simulink model "Speed_Controller"  (R2019b)
settings: Solver=VariableStepAuto  StartTime=0.0  StopTime=10.0  RelTol=1e-3
values from neighbouring files (symbols this model uses):
  B = 1/3*Te_n*1/w_b    (= 1.3022339824)    [tram.m]
  e_n = Ks*ie_max*w_b    (= 540)    [tram.m]
  g = 9.81    [tram.m]
  ie_max = 1    [tram.m]
  J = m_t*r_whl^2    (= 73.2506615098)    [tram.m]
  kb_e = 1/tau_e    (= 1)    [tram.m]
  kb_spd = 1/tau_s    (= 5)    [tram.m]
  Kie = Ci_e.Ki    [tram.m]
  Kim = Cm.Ki    [tram.m]
  Kpe = Ci_e.Kp    [tram.m]
  Kpm = Cm.Kp    [tram.m]
  Ks = v_line*eta/(ie_max*w_b)    (= 1.71974522293)    [tram.m]
  Le = tau_e*Re    (= 120)    [tram.m]
  m_t = m_train + m_load    (= 26000)    [tram.m]
  r_whl = s_b/w_b*10/36    (= 0.0530785562633)    [tram.m]
  Re = ve_max/ie_max    (= 120)    [tram.m]
  w_b = 314    [tram.m]
undefined symbols (not defined in the file or in its folder): sigbuilder_block
settings Model: Creator=hassancurrimbhoy  LastModifiedBy=hassancurrimbhoy

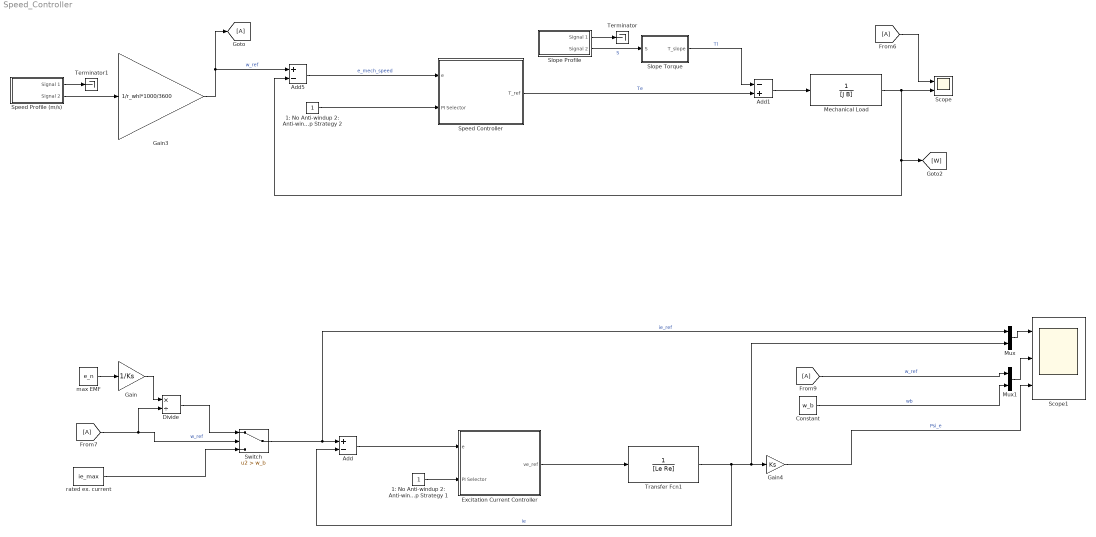
== system Speed_Controller ==
  1: No Anti-windup 2: Anti-windup Stragtegy 1 3: Anti-windup Strategy 2 : Constant
  1: No Anti-windup 2: Anti-windup Strategy 1 3: Anti-windup Strategy 1 : Constant
  Add : Sum  Inputs=+-
  Add1 : Sum  Inputs=-+
  Add5 : Sum  Inputs=+-
  Constant : Constant  Value=w_b
  Divide : Product  Inputs=*/
  Excitation Current Controller : Subsystem
  Gain : Gain  Gain=1/Ks
  Gain3 : Gain  Gain=1/r_whl*1000/3600
  Gain4 : Gain  Gain=Ks
  Mechanical Load : TransferFcn  Denominator=[J B]
  Mux : Mux  Inputs=2
  Mux1 : Mux  Inputs=2
  Scope : Scope  NumInputPorts=2
  Scope1 : Scope  NumInputPorts=3
  Slope Profile : Subsystem  Tag=STV Subsys  LoadFcn=sigbuilder_block('load');  StartFcn=sigbuilder_block('start');  StopFcn=sigbuilder_block('stop');  ClipboardFcn=sigbuilder_block('clipboard');  mask(Sigbuilder block){tuvar=[0:10]}
      mask help: Simulink:masks:SigbuilderBlock_MD
      mask init:
      | if ~strcmp(get_param(bdroot(gcbh),'SimulationStatus'),'stopped') tuvar = sigbuilder_block('maskInit'); end
      settings: CopyFcn=sigbuilder_block('copy');  DeleteFcn=sigbuilder_block('delete');  ModelCloseFcn=sigbuilder_block('modelClose');  PreSaveFcn=sigbuilder_block('preSave');  PauseFcn=sigbuilder_block('pause');  ContinueFcn=sigbuilder_block('continue');  NameChangeFcn=sigbuilder_block('namechange');  OpenFcn=sigbuilder_block('open',[437.6 199.2 550.4 400 ]);  CloseFcn=sigbuilder_block('close');
      mask Display: plot(0, 0, 100, 100,[2, 2, 32, 32, 2], [68, 8, 8, 68, 68],[32, 2], [38, 38], [32, 19, 2],[53, 60, 44], [32, 17, 17, 2],[16, 16, 31, 31]);txt = getActiveGroup(gcbh);text(2, 100, txt,'verticalAlignment', 'top');
  Slope Torque : Subsystem
  Speed Controller : Subsystem
  Speed Profile (m/s) : Subsystem  Tag=STV Subsys  LoadFcn=sigbuilder_block('load');  StartFcn=sigbuilder_block('start');  StopFcn=sigbuilder_block('stop');  ClipboardFcn=sigbuilder_block('clipboard');  mask(Sigbuilder block){tuvar=[0:10]}
      mask help: Simulink:masks:SigbuilderBlock_MD
      mask init:
      | if ~strcmp(get_param(bdroot(gcbh),'SimulationStatus'),'stopped') tuvar = sigbuilder_block('maskInit'); end
      settings: CopyFcn=sigbuilder_block('copy');  DeleteFcn=sigbuilder_block('delete');  ModelCloseFcn=sigbuilder_block('modelClose');  PreSaveFcn=sigbuilder_block('preSave');  PauseFcn=sigbuilder_block('pause');  ContinueFcn=sigbuilder_block('continue');  NameChangeFcn=sigbuilder_block('namechange');  OpenFcn=sigbuilder_block('open',[437.6 199.2 550.4 400 ]);  CloseFcn=sigbuilder_block('close');
      mask Display: plot(0, 0, 100, 100,[2, 2, 32, 32, 2], [68, 8, 8, 68, 68],[32, 2], [38, 38], [32, 19, 2],[53, 60, 44], [32, 17, 17, 2],[16, 16, 31, 31]);txt = getActiveGroup(gcbh);text(2, 100, txt,'verticalAlignment', 'top');
  Switch : Switch  Criteria=u2 > Threshold  Threshold=w_b
  Terminator : Terminator
  Terminator1 : Terminator
  Transfer Fcn1 : TransferFcn  Denominator=[Le Re]
  max EMF : Constant  Value=e_n
  rated ex. current : Constant  Value=ie_max
  wires:
  Mux1/1 -> Scope1/2
  Gain4/1 -> Scope1/3  "Psi_e"
  1: No Anti-windup 2: Anti-windup Stragtegy 1 3: Anti-windup Strategy 2/1 -> Speed Controller/2(PI Selector)
  [A] -> Mux1/1  "w_ref"
  Add1/1 -> Mechanical Load/1
  [A] -> Divide/2, Switch/2  "w_ref"
  Constant/1 -> Mux1/2  "wb"
  Gain3/1 -> Add5/1, [A]  "w_ref"
  Gain/1 -> Divide/1
  Mechanical Load/1 -> Add5/2, [W], Scope/2
  max EMF/1 -> Gain/1
  Add5/1 -> Speed Controller/1(e)  "e_mech_speed"
  Slope Profile/1(Signal 1) -> Terminator/1
  Transfer Fcn1/1 -> Mux/2, Gain4/1, Add/2  "ie"
  rated ex. current/1 -> Switch/3
  1: No Anti-windup 2: Anti-windup Strategy 1 3: Anti-windup Strategy 1/1 -> Excitation Current Controller/2("PI Selector ")
  Excitation Current Controller/1("ve_ref ") -> Transfer Fcn1/1
  Divide/1 -> Switch/1
  Mux/1 -> Scope1/1
  Add/1 -> Excitation Current Controller/1(e)
  [A] -> Scope/1
  Slope Profile/2(Signal 2) -> Slope Torque/1(S)  "S"
  Speed Controller/1("T_ref ") -> Add1/2  "Te"
  Speed Profile (m/s)/1(Signal 1) -> Terminator1/1
  Switch/1 -> Mux/1, Add/1  "ie_ref"
  Slope Torque/1(T_slope) -> Add1/1  "Tl"
  Speed Profile (m/s)/2(Signal 2) -> Gain3/1

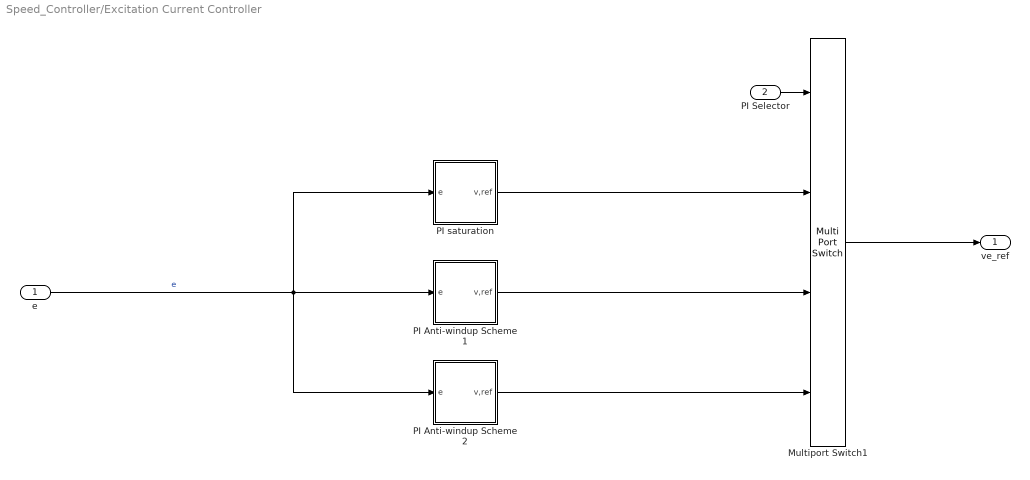
== system Speed_Controller/Excitation Current Controller ==
  e : Inport
  "PI Selector " : Inport  Port=2
  Multiport Switch1 : MultiPortSwitch
  PI Anti-windup Scheme 1 : Subsystem
  PI Anti-windup Scheme 2 : Subsystem
  PI saturation : Subsystem
  "ve_ref " : Outport
  wires:
  PI saturation/1(v,ref) -> Multiport Switch1/2
  PI Anti-windup Scheme 2/1(v,ref) -> Multiport Switch1/4
  e/1 -> PI saturation/1(e), PI Anti-windup Scheme 1/1(e), PI Anti-windup Scheme 2/1(e)  "e"
  PI Anti-windup Scheme 1/1(v,ref) -> Multiport Switch1/3
  "PI Selector "/1 -> Multiport Switch1/1
  Multiport Switch1/1 -> "ve_ref "/1

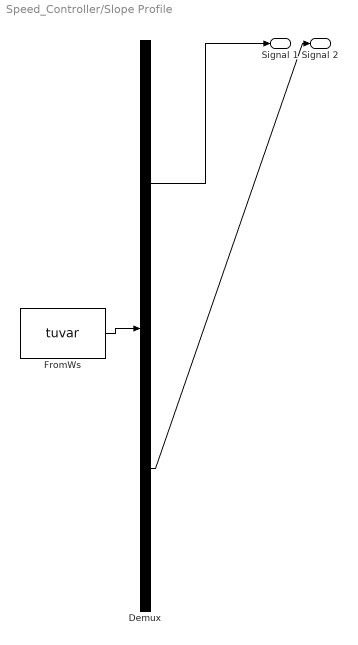
== system Speed_Controller/Slope Profile ==
  Demux : Demux  Tag=STV Demux  Outputs=2
  FromWs : FromWorkspace  Tag=STV FromWs  VariableName=tuvar  SampleTime=0
      SigBuilderData=|
      | common.afterFinalStr = 'Extrapolate'
      | common.sampleTime = 0
      | dataSet.timeRange = [0 10]
      | dataSet.name = 'Group 1'
      | sbobj.Groups.Name = 'Group 1'
      | sbobj.Groups.Signals(1).Name = 'Signal 1'
      | sbobj.Groups.Signals(1).XData = [0 4 4 6 6 10]
      | sbobj.Groups.Signals(1).YData = [0 0 1 1 0 0]
      | sbobj.Groups.Signals(2).Name = 'Signal 2'
      | sbobj.Groups.Signals(2).XData = [0 1 2 3 3 4 4 5 6 7 8 8 9 9 10]
      | sbobj.Groups.Signals(2).YData = [0 0 0 0 5 5 0 0 0 0 0 -5 -5 0 0]
  Signal 1 : Outport  Tag=STV Outport
  Signal 2 : Outport  Tag=STV Outport  Port=2
  wires:
  Demux/1 -> Signal 1/1
  FromWs/1 -> Demux/1
  Demux/2 -> Signal 2/1

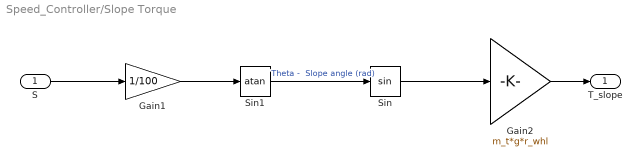
== system Speed_Controller/Slope Torque ==
  S : Inport
  Gain1 : Gain  Gain=1/100
  Gain2 : Gain  Gain=m_t*g*r_whl
  Sin : Trigonometry
  Sin1 : Trigonometry  Operator=atan
  T_slope : Outport
  wires:
  Sin/1 -> Gain2/1
  S/1 -> Gain1/1
  Sin1/1 -> Sin/1  "Theta -  Slope angle (rad)"
  Gain2/1 -> T_slope/1
  Gain1/1 -> Sin1/1

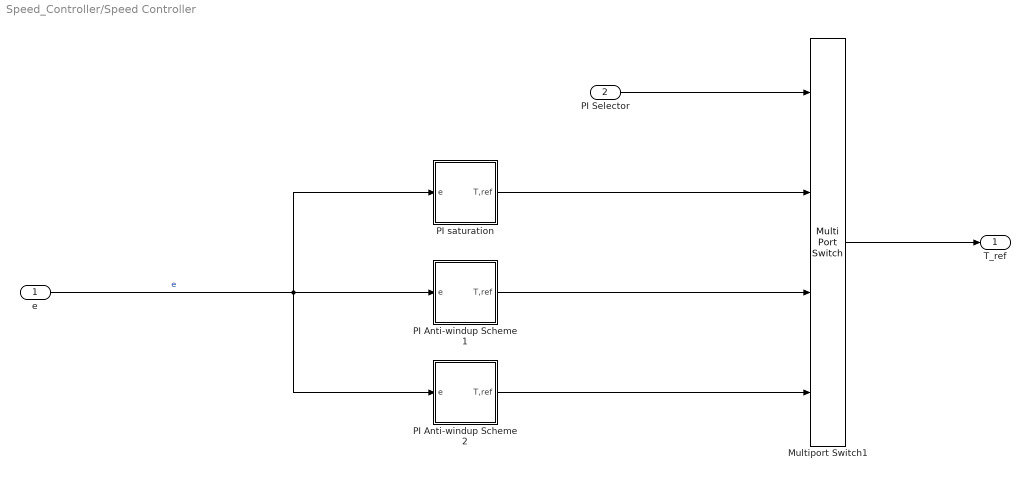
== system Speed_Controller/Speed Controller ==
  e : Inport
  PI Selector : Inport  Port=2
  Multiport Switch1 : MultiPortSwitch
  PI Anti-windup Scheme 1 : Subsystem
  PI Anti-windup Scheme 2 : Subsystem
  PI saturation : Subsystem
  "T_ref " : Outport
  wires:
  PI Anti-windup Scheme 1/1(T,ref) -> Multiport Switch1/3
  e/1 -> PI saturation/1(e), PI Anti-windup Scheme 1/1(e), PI Anti-windup Scheme 2/1(e)  "e"
  Multiport Switch1/1 -> "T_ref "/1
  PI saturation/1(T,ref) -> Multiport Switch1/2
  PI Selector/1 -> Multiport Switch1/1
  PI Anti-windup Scheme 2/1(T,ref) -> Multiport Switch1/4

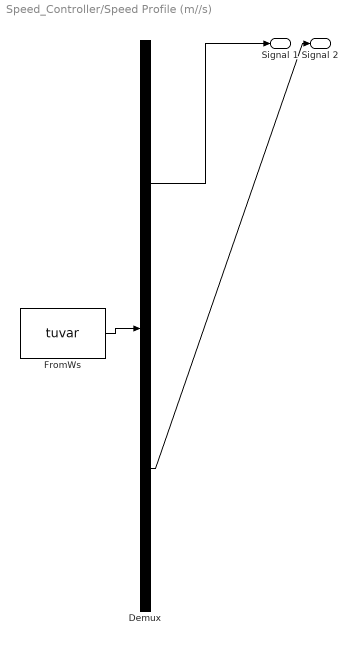
== system Speed_Controller/Speed Profile (m//s) ==
  Demux : Demux  Tag=STV Demux  Outputs=2
  FromWs : FromWorkspace  Tag=STV FromWs  VariableName=tuvar  SampleTime=0
      SigBuilderData=|
      | common.afterFinalStr = 'Extrapolate'
      | common.sampleTime = 0
      | dataSet.timeRange = [0 10]
      | dataSet.name = 'Group 1'
      | sbobj.Groups.Name = 'Group 1'
      | sbobj.Groups.Signals(1).Name = 'Signal 1'
      | sbobj.Groups.Signals(1).XData = [0 1 1 2 2 10]
      | sbobj.Groups.Signals(1).YData = [0 0 35 35 60 0]
      | sbobj.Groups.Signals(2).Name = 'Signal 2'
      | sbobj.Groups.Signals(2).XData = [0 1 1 2 2 3 4 4 5 6 6 7 8 9 9 10]
      | sbobj.Groups.Signals(2).YData = [0 0 35 35 60 60 60 75 75 75 60 60 60 60 35 35]
  Signal 1 : Outport  Tag=STV Outport
  Signal 2 : Outport  Tag=STV Outport  Port=2
  wires:
  Demux/1 -> Signal 1/1
  FromWs/1 -> Demux/1
  Demux/2 -> Signal 2/1

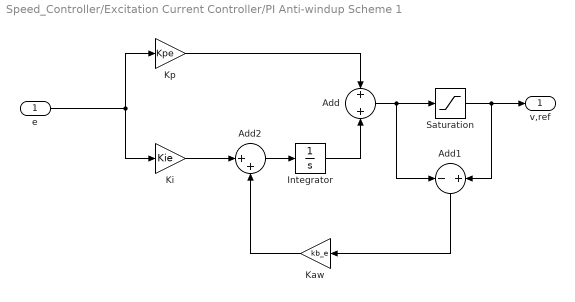
== system Speed_Controller/Excitation Current Controller/PI Anti-windup Scheme 1 ==
  e : Inport
  Add : Sum
  Add1 : Sum  Inputs=-+
  Add2 : Sum  Inputs=|++
  Integrator : Integrator
  Kaw : Gain  Gain=kb_e
  Ki : Gain  Gain=Kie
  Kp : Gain  Gain=Kpe
  Saturation : Saturate  UpperLimit=1  LowerLimit=-1
  v,ref : Outport
  wires:
  Ki/1 -> Add2/1
  Kp/1 -> Add/1
  Add/1 -> Add1/1, Saturation/1
  Integrator/1 -> Add/2
  e/1 -> Ki/1, Kp/1
  Saturation/1 -> Add1/2, v,ref/1
  Add2/1 -> Integrator/1
  Add1/1 -> Kaw/1
  Kaw/1 -> Add2/2

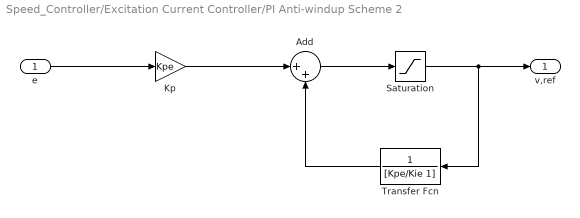
== system Speed_Controller/Excitation Current Controller/PI Anti-windup Scheme 2 ==
  e : Inport
  Add : Sum  Inputs=|++
  Kp : Gain  Gain=Kpe
  Saturation : Saturate  UpperLimit=1  LowerLimit=-1
  Transfer Fcn : TransferFcn  Denominator=[Kpe/Kie 1]
  v,ref : Outport
  wires:
  Kp/1 -> Add/1
  e/1 -> Kp/1
  Add/1 -> Saturation/1
  Transfer Fcn/1 -> Add/2
  Saturation/1 -> Transfer Fcn/1, v,ref/1

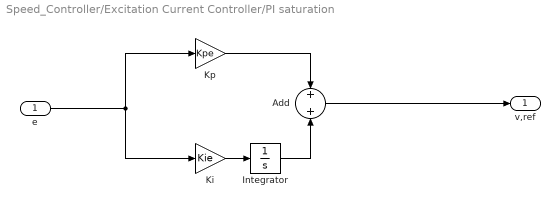
== system Speed_Controller/Excitation Current Controller/PI saturation ==
  e : Inport
  Add : Sum
  Integrator : Integrator
  Ki : Gain  Gain=Kie
  Kp : Gain  Gain=Kpe
  v,ref : Outport
  wires:
  Ki/1 -> Integrator/1
  Kp/1 -> Add/1
  Integrator/1 -> Add/2
  e/1 -> Ki/1, Kp/1
  Add/1 -> v,ref/1

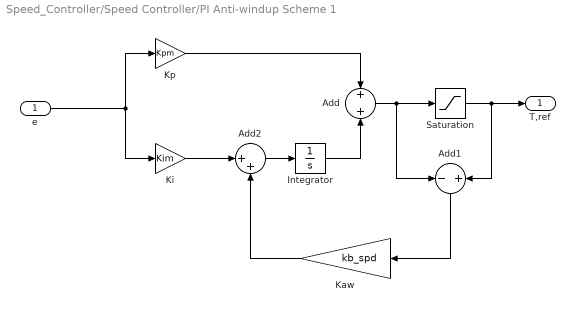
== system Speed_Controller/Speed Controller/PI Anti-windup Scheme 1 ==
  e : Inport
  Add : Sum
  Add1 : Sum  Inputs=-+
  Add2 : Sum  Inputs=|++
  Integrator : Integrator
  Kaw : Gain  Gain=kb_spd
  Ki : Gain  Gain=Kim
  Kp : Gain  Gain=Kpm
  Saturation : Saturate
  T,ref : Outport
  wires:
  Ki/1 -> Add2/1
  Kp/1 -> Add/1
  Add/1 -> Add1/1, Saturation/1
  Integrator/1 -> Add/2
  e/1 -> Ki/1, Kp/1
  Saturation/1 -> Add1/2, T,ref/1
  Add2/1 -> Integrator/1
  Add1/1 -> Kaw/1
  Kaw/1 -> Add2/2

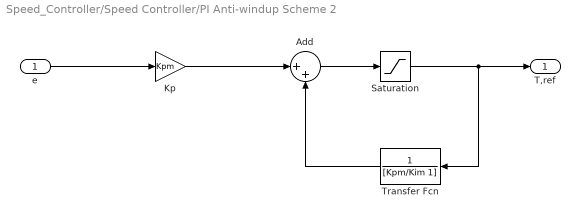
== system Speed_Controller/Speed Controller/PI Anti-windup Scheme 2 ==
  e : Inport
  Add : Sum  Inputs=|++
  Kp : Gain  Gain=Kpm
  Saturation : Saturate  UpperLimit=45  LowerLimit=-45
  Transfer Fcn : TransferFcn  Denominator=[Kpm/Kim 1]
  T,ref : Outport
  wires:
  Kp/1 -> Add/1
  e/1 -> Kp/1
  Saturation/1 -> Transfer Fcn/1, T,ref/1
  Add/1 -> Saturation/1
  Transfer Fcn/1 -> Add/2

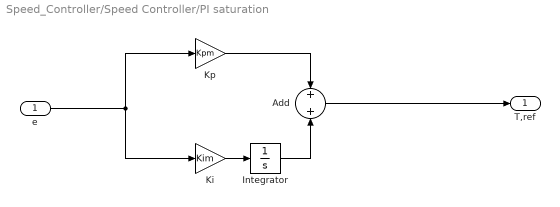
== system Speed_Controller/Speed Controller/PI saturation ==
  e : Inport
  Add : Sum
  Integrator : Integrator
  Ki : Gain  Gain=Kim
  Kp : Gain  Gain=Kpm
  T,ref : Outport
  wires:
  Ki/1 -> Integrator/1
  Kp/1 -> Add/1
  Integrator/1 -> Add/2
  e/1 -> Ki/1, Kp/1
  Add/1 -> T,ref/1
